simulink model "PDGravityCompensationOS"  (R2020b)
settings: Solver=VariableStepAuto  StartTime=0.0  StopTime=4  RelTol=1e-3
values from neighbouring files (symbols this model uses):
  Kd = diag([50 50 50 1 1 1])    [params.m]
  Kp = diag([700 700 700 1 1 1])    [params.m]
  xd = Kinematics([t1,d2,d3], param)    [params.m]
settings Model: Creator=andre  LastModifiedBy=filippo

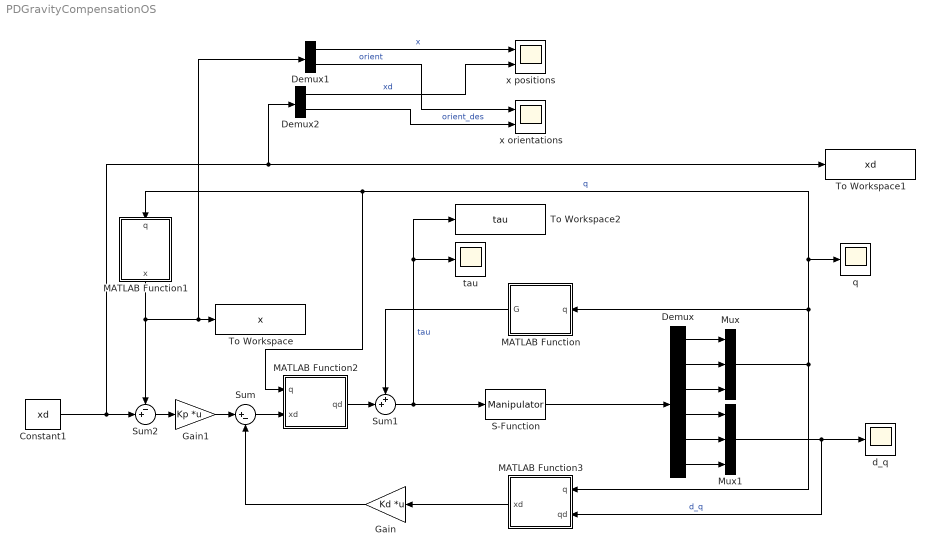
== system PDGravityCompensationOS ==
  Constant1 : Constant  Value=xd
  Demux : Demux  Outputs=6
  Demux1 : Demux  Outputs=2
  Demux2 : Demux  Outputs=2
  Gain : Gain  Gain=Kd  Multiplication=Matrix(K*u)
  Gain1 : Gain  Gain=Kp  Multiplication=Matrix(K*u)
  MATLAB Function : MATLAB Function  TreatAsAtomicUnit=on
  MATLAB Function1 : MATLAB Function  TreatAsAtomicUnit=on
  MATLAB Function2 : MATLAB Function  TreatAsAtomicUnit=on
  MATLAB Function3 : MATLAB Function  TreatAsAtomicUnit=on
  Mux : Mux  Inputs=3
  Mux1 : Mux  Inputs=3
  S-Function : S-Function  FunctionName=Manipulator  Parameters=param  SFunctionDeploymentMode=off  EnableBusSupport=off
  Sum : Sum  Inputs=|+-
  Sum1 : Sum  Inputs=++|
  Sum2 : Sum  Inputs=-+|
  To Workspace : ToWorkspace  VariableName=x  SaveFormat=Timeseries  SampleTime=-1
  To Workspace1 : ToWorkspace  VariableName=xd  SaveFormat=Timeseries  SampleTime=-1
  To Workspace2 : ToWorkspace  VariableName=tau  SaveFormat=Timeseries  SampleTime=-1
  d_q : Scope
  q : Scope
  tau : Scope
  x orientations : Scope  NumInputPorts=2
  x positions : Scope  NumInputPorts=2
  wires:
  Gain1/1 -> Sum/1
  S-Function/1 -> Demux/1
  Demux/3 -> Mux/3
  Demux/2 -> Mux/2
  Demux/1 -> Mux/1
  Demux/4 -> Mux1/1
  Demux/5 -> Mux1/2
  Demux/6 -> Mux1/3
  Mux/1 -> q/1, MATLAB Function2/1(q), MATLAB Function1/1(q), MATLAB Function/1(q), MATLAB Function3/1(q)  "q"
  Sum1/1 -> To Workspace2/1, tau/1, S-Function/1  "tau"
  Gain/1 -> Sum/2
  Sum2/1 -> Gain1/1
  Mux1/1 -> MATLAB Function3/2(qd), d_q/1  "d_q"
  Constant1/1 -> Sum2/2, Demux2/1, To Workspace1/1
  MATLAB Function1/1(x) -> Sum2/1, Demux1/1, To Workspace/1
  MATLAB Function2/1(qd) -> Sum1/2
  MATLAB Function3/1(xd) -> Gain/1
  Sum/1 -> MATLAB Function2/2(xd)
  Demux1/1 -> x positions/1  "x"
  Demux2/1 -> x positions/2  "xd"
  Demux1/2 -> x orientations/1  "orient"
  Demux2/2 -> x orientations/2  "orient_des"
  MATLAB Function/1(G) -> Sum1/1

== matlab function PDGravityCompensationOS/MATLAB Function ==
  data: q input; G output; param parameter
function G = Gravity(q, param)
    G = G_Lagrangian(q,param);
end

== matlab function PDGravityCompensationOS/MATLAB Function2 ==
  data: q input; xd input; qd output; param parameter
function qd = JaT(q, xd, param)
    Ja = AnalyticalJacobian(q,param);
    qd = Ja' * xd;
end

== matlab function PDGravityCompensationOS/MATLAB Function3 ==
  data: q input; qd input; xd output; param parameter
function xd = Ja(q, qd, param)
    Ja = AnalyticalJacobian(q,param);
    xd = Ja * qd;
end

== matlab function PDGravityCompensationOS/MATLAB Function1 ==
  data: q input; x output; param parameter
function x = Kin(q,param)
    x = Kinematics(q,param);
end
